simulink model "joe_fft"  (R2022b)
settings: Solver=FixedStepDiscrete  StartTime=0.0  StopTime=48*FFTLength/FrameSize  RelTol=1e-3
InitFcn:
  | FFTLength = 2^9;
  | Fs = 1*2e6;
  | FrameSize = 8;
  | ValidPattern = [1, 0];
libraries: hdlsllib x3, dsphdlsigops2 x1
settings Model: DataTypeOverride=Off  Creator=The MathWorks, Inc.  LastModifiedBy=jwbie
settings SolverCC: AlgebraicLoopSolver=TrustRegion  AutoInsertRateTranBlk=on  MaxZcPerStep=1
settings DataIOCC: SaveOutput=off  SaveTime=off  ReturnWorkspaceOutputs=off
settings OptimizationCC: BlockReduction=off  ConditionallyExecuteInputs=off  DefaultParameterBehavior=Inlined
settings DebuggingCC: AlgebraicLoopMsg=error  SingleTaskRateTransMsg=error  UnconnectedInputMsg=warning  UnconnectedOutputMsg=warning  UnconnectedLineMsg=warning  SFMachineParentedDataDiag=warning  ArithmeticOperatorsInVariantConditions=warning
settings HardwareCC: ProdBitPerPointer=32  ProdBitPerSizeT=32  ProdBitPerPtrDiffT=32  ProdLargestAtomicFloat=None  ProdIntDivRoundTo=Undefined  ProdEndianess=Unspecified  ProdWordSize=32  ProdHWDeviceType=ASIC/FPGA->ASIC/FPGA  ProdEqTarget=off
settings ModelReferenceCC: EnableRefExpFcnMdlSchedulingChecks=on
settings SFSimCC: SimUseLocalCustomCode=off  CustomCodeUndefinedFunction=UseInterfaceOnly
settings RTWCC: RTWUseLocalCustomCode=off  DLArmComputeVersion=19.05
settings CodeAppCC: StateflowObjectComments=on

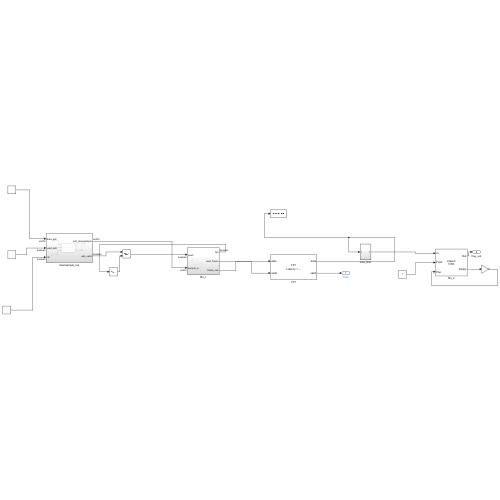
[thumbnail: Simulink's stored preview of the top-level diagram]
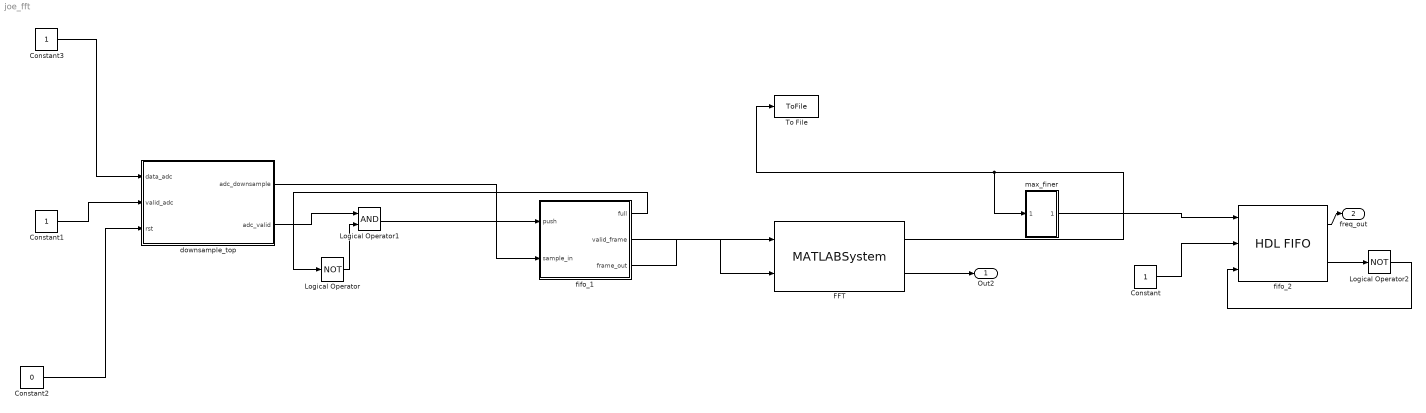
== system joe_fft ==
  Constant : Constant  OutDataTypeStr=boolean  SampleTime=8
  Constant1 : Constant  OutDataTypeStr=boolean  SampleTime=-1
  Constant2 : Constant  Value=0  OutDataTypeStr=boolean  SampleTime=-1
  Constant3 : Constant  OutDataTypeStr=uint16  SampleTime=1
  FFT : MATLABSystem  System=dsphdl.FFT  FFTLength=16  Architecture=Streaming Radix 2^2  ComplexMultiplication=Use 4 multipliers and 2 adders  BitReversedOutput=off  BitReversedInput=off  Normalize=off  SimulateUsing=Code generation  RoundingMethod=Floor  ResetInputPort=off  StartOutputPort=off  EndOutputPort=off
      settings: LibrarySourceBlock=dsphdlxfrm2/FFT
      mask Type: FFT
      mask Display:
      | disp(['FFT' char(10) 'Latency = 34']);
      | port_label('input',1,'data');
      | port_label('input',2,'valid');
      | port_label('output',1,'data');
      | port_label('output',2,'valid');
  Logical Operator : Logic  Operator=NOT  AllPortsSameDT=off  OutDataTypeStr=boolean
  Logical Operator1 : Logic  AllPortsSameDT=off  OutDataTypeStr=boolean
  Logical Operator2 : Logic  Operator=NOT  IconShape=distinctive  AllPortsSameDT=off  OutDataTypeStr=boolean
  To File : ToFile  SaveFormat=Timeseries
  downsample_top : Subsystem
  fifo_1 : Subsystem
  fifo_2 : hdlsllib/HDL RAMs/HDL FIFO  fifo_size=1024  mode=Classic  ratio=1  push_msg=Warning  pop_msg=Warning  show_empty=on  show_full=off  show_num=off  LabelModeActiveChoice_Mode=Classic  rst_port=off
  max_finer : Subsystem
  Out2 : Outport  VectorParamsAs1DForOutWhenUnconnected=off
  freq_out : Outport  Port=2  VectorParamsAs1DForOutWhenUnconnected=off
  wires:
  downsample_top/1(adc_downsample) -> fifo_1/2(sample_in)
  downsample_top/2(adc_valid) -> Logical Operator1/1
  Logical Operator/1 -> Logical Operator1/2
  fifo_1/1(full) -> Logical Operator/1
  Logical Operator1/1 -> fifo_1/1(push)
  Constant2/1 -> downsample_top/3(rst)
  Constant1/1 -> downsample_top/2(valid_adc)
  FFT/2 -> Out2/1
  fifo_1/2(valid_frame) -> FFT/2
  FFT/1 -> max_finer/1(In1), To File/1
  fifo_1/3(frame_out) -> FFT/1
  Constant/1 -> fifo_2/2
  fifo_2/2 -> Logical Operator2/1
  Logical Operator2/1 -> fifo_2/3
  Constant3/1 -> downsample_top/1(data_adc)
  fifo_2/1 -> freq_out/1
  max_finer/1(Out1) -> fifo_2/1

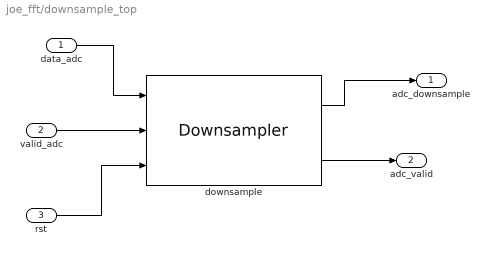
== system joe_fft/downsample_top ==
  data_adc : Inport  OutDataTypeStr=uint16
  valid_adc : Inport  Port=2  OutDataTypeStr=boolean
  rst : Inport  Port=3  OutDataTypeStr=boolean
  downsample : dsphdlsigops2/Downsampler  DownsampleFactor=13  SampleOffset=0  SimulateUsing=Code generation  ResetInputPort=on
  adc_downsample : Outport  OutDataTypeStr=uint16  VectorParamsAs1DForOutWhenUnconnected=off
  adc_valid : Outport  Port=2  OutDataTypeStr=boolean  VectorParamsAs1DForOutWhenUnconnected=off
  wires:
  data_adc/1 -> downsample/1
  rst/1 -> downsample/3
  valid_adc/1 -> downsample/2
  downsample/2 -> adc_valid/1
  downsample/1 -> adc_downsample/1

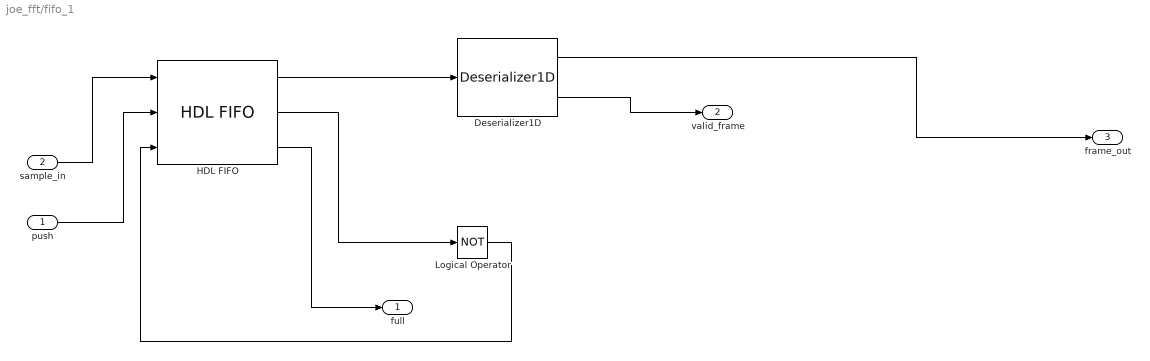
== system joe_fft/fifo_1 ==
  push : Inport  OutDataTypeStr=boolean
  sample_in : Inport  Port=2  OutDataTypeStr=uint16
  Deserializer1D : hdlsllib/HDL Operations/Deserializer1D  Ratio=8/1  IdleCycles=0  InitialCondition=0  startIn=off  validIn=off  validOut=on  inputDataDimensions=-1  inputSampleTime=1  inputSignalType=auto
  HDL FIFO : hdlsllib/HDL RAMs/HDL FIFO  fifo_size=10  mode=Classic  ratio=1  push_msg=Warning  pop_msg=Warning  show_empty=on  show_full=on  show_num=off  LabelModeActiveChoice_Mode=Classic  rst_port=off
  Logical Operator : Logic  Operator=NOT  IconShape=distinctive  AllPortsSameDT=off  OutDataTypeStr=boolean
  full : Outport  OutDataTypeStr=boolean  VectorParamsAs1DForOutWhenUnconnected=off
  valid_frame : Outport  Port=2  VectorParamsAs1DForOutWhenUnconnected=off
  frame_out : Outport  Port=3  VectorParamsAs1DForOutWhenUnconnected=off
  wires:
  sample_in/1 -> HDL FIFO/1
  HDL FIFO/3 -> full/1
  push/1 -> HDL FIFO/2
  HDL FIFO/2 -> Logical Operator/1
  Logical Operator/1 -> HDL FIFO/3
  HDL FIFO/1 -> Deserializer1D/1
  Deserializer1D/2 -> valid_frame/1
  Deserializer1D/1 -> frame_out/1

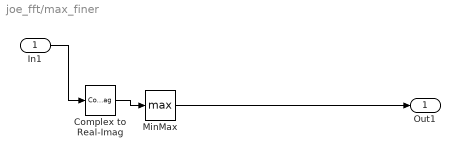
== system joe_fft/max_finer ==
  In1 : Inport
  Complex to Real-Imag : ComplexToRealImag  Output=Real
  MinMax : MinMax  Function=max  OutDataTypeStr=uint16
  Out1 : Outport
  wires:
  Complex to Real-Imag/1 -> MinMax/1
  In1/1 -> Complex to Real-Imag/1
  MinMax/1 -> Out1/1
